simulink model "gm_spike_detection"  (R2020a)
settings: Solver=FixedStepDiscrete  StartTime=0.0  StopTime=840000  RelTol=1e-3
undefined symbols (not defined in the file or in its folder): Newton, Raphson
libraries: hdlsllib x8, simulink x4
settings Model: FPTRunName=FPA_Reference  PacingRate=40  Creator=BuccelliLab  LastModifiedBy=diflo
settings SolverCC: AutoInsertRateTranBlk=on  MinimalZcImpactIntegration=on
settings DataIOCC: LimitDataPoints=on  SaveOutput=off  SaveTime=off  ReturnWorkspaceOutputs=off
settings OptimizationCC: BlockReduction=off  ConditionallyExecuteInputs=off  DefaultParameterBehavior=Inlined  LifeSpan=inf
settings DebuggingCC: SignalRangeChecking=warning  ReadBeforeWriteMsg=DisableAll  WriteAfterWriteMsg=DisableAll  WriteAfterReadMsg=DisableAll  AlgebraicLoopMsg=error  InheritedTsInSrcMsg=none  MultiTaskDSMMsg=none  SingleTaskRateTransMsg=error  ParameterDowncastMsg=warning  ParameterOverflowMsg=warning  AllowSymbolicDim=off  StrictBusMsg=ErrorOnBusTreatedAsVector  SFUnexpectedBacktrackingDiag=warning  SFNoUnconditionalDefaultTransitionDiag=warning  SFExecutionAtInitializationDiag=none  ArithmeticOperatorsInVariantConditions=warning
settings HardwareCC: ProdBitPerPointer=32  ProdBitPerSizeT=32  ProdBitPerPtrDiffT=32  ProdLargestAtomicFloat=None  ProdIntDivRoundTo=Undefined  ProdEndianess=Unspecified  ProdWordSize=32  ProdHWDeviceType=ASIC/FPGA->ASIC/FPGA  TargetBitPerPointer=64  TargetBitPerSizeT=64  TargetBitPerPtrDiffT=64  TargetLongLongMode=on  TargetIntDivRoundTo=Zero  TargetEndianess=LittleEndian  TargetWordSize=64  TargetHWDeviceType=Custom Processor->MATLAB Host Computer  ProdEqTarget=off
settings ModelReferenceCC: UpdateModelReferenceTargets=IfOutOfDate
settings SFSimCC: SFSimEcho=off  SimUseLocalCustomCode=off  CustomCodeUndefinedFunction=UseInterfaceOnly
settings RTWCC: RTWUseLocalCustomCode=off
settings CodeAppCC: StateflowObjectComments=on
settings GRTTargetCC: TargetLangStandard=C89/C90 (ANSI)
settings ConfigComp: CovScope=ReferencedModels  CovMetricSettings=dw  CovHtmlReporting=on  CovSaveCumulativeToWorkspaceVar=on  CovSaveSingleToWorkspaceVar=on  CovExternalEMLEnable=off  CovSFcnEnable=off

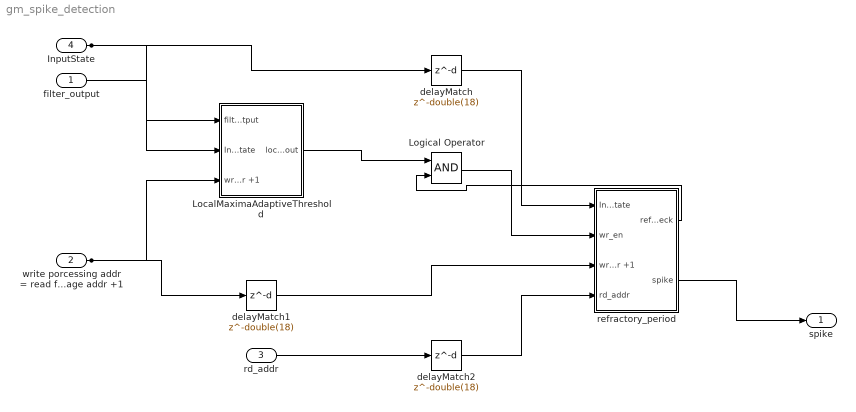
== system gm_spike_detection ==
  filter_output : Inport  OutDataTypeStr=uint16  PortDimensions=1  SampleTime=1
  write porcessing addr = read from storage addr +1 : Inport  Port=2  OutDataTypeStr=fixdt(0, 9, 0)  PortDimensions=1  SampleTime=1
  rd_addr : Inport  Port=3  OutDataTypeStr=fixdt(0, 9, 0)  PortDimensions=1  SampleTime=1
  InputState : Inport  Port=4  OutDataTypeStr=boolean  PortDimensions=1  SampleTime=1
  LocalMaximaAdaptiveThreshold : Subsystem
  Logical Operator : Logic  AllPortsSameDT=off  OutDataTypeStr=boolean  SampleTime=1
  delayMatch : Delay  DelayLength=double(18)  InitialCondition=0  SampleTime=1
  delayMatch1 : Delay  DelayLength=double(18)  InitialCondition=0  SampleTime=1
  delayMatch2 : Delay  DelayLength=double(18)  InitialCondition=0  SampleTime=1
  refractory_period : Subsystem
  spike : Outport  OutDataTypeStr=uint16  PortDimensions=1  SampleTime=[1,0]
  wires:
  filter_output/1 -> LocalMaximaAdaptiveThreshold/1(filter_output)
  delayMatch1/1 -> refractory_period/3(write porcessing addr = read from storage addr +1)
  delayMatch2/1 -> refractory_period/4(rd_addr)
  delayMatch/1 -> refractory_period/1(InputState)
  LocalMaximaAdaptiveThreshold/1(local_maxima_out) -> Logical Operator/1
  InputState/1 -> delayMatch/1, LocalMaximaAdaptiveThreshold/2(InputState)
  write porcessing addr = read from storage addr +1/1 -> delayMatch1/1, LocalMaximaAdaptiveThreshold/3(write porcessing addr = read from storage addr +1)
  rd_addr/1 -> delayMatch2/1
  Logical Operator/1 -> refractory_period/2(wr_en)
  refractory_period/1(refractory_check) -> Logical Operator/2
  refractory_period/2(spike) -> spike/1

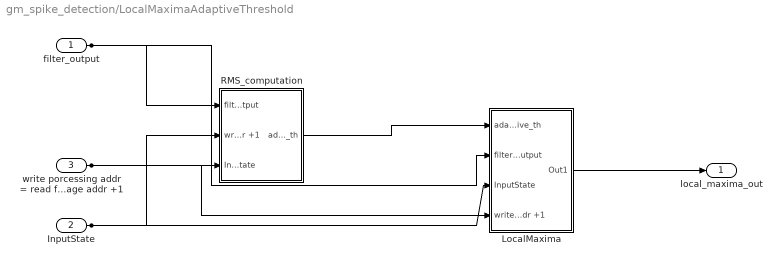
== system gm_spike_detection/LocalMaximaAdaptiveThreshold ==
  filter_output : Inport  OutDataTypeStr=uint16  PortDimensions=1  SampleTime=1
  InputState : Inport  Port=2  OutDataTypeStr=boolean  PortDimensions=1  SampleTime=1
  write porcessing addr = read from storage addr +1 : Inport  Port=3  OutDataTypeStr=fixdt(0, 9, 0)  PortDimensions=1  SampleTime=1
  LocalMaxima : Subsystem
  RMS_computation : Subsystem
  local_maxima_out : Outport
  wires:
  LocalMaxima/1(Out1) -> local_maxima_out/1
  RMS_computation/1(adaptive_th) -> LocalMaxima/1(adaptive_th)
  filter_output/1 -> LocalMaxima/2(filter_output), RMS_computation/1(filter_output)
  InputState/1 -> LocalMaxima/3(InputState), RMS_computation/3(InputState)
  write porcessing addr = read from storage addr +1/1 -> LocalMaxima/4(write porcessing addr = read from storage addr +1), RMS_computation/2(write porcessing addr = read from storage addr +1)

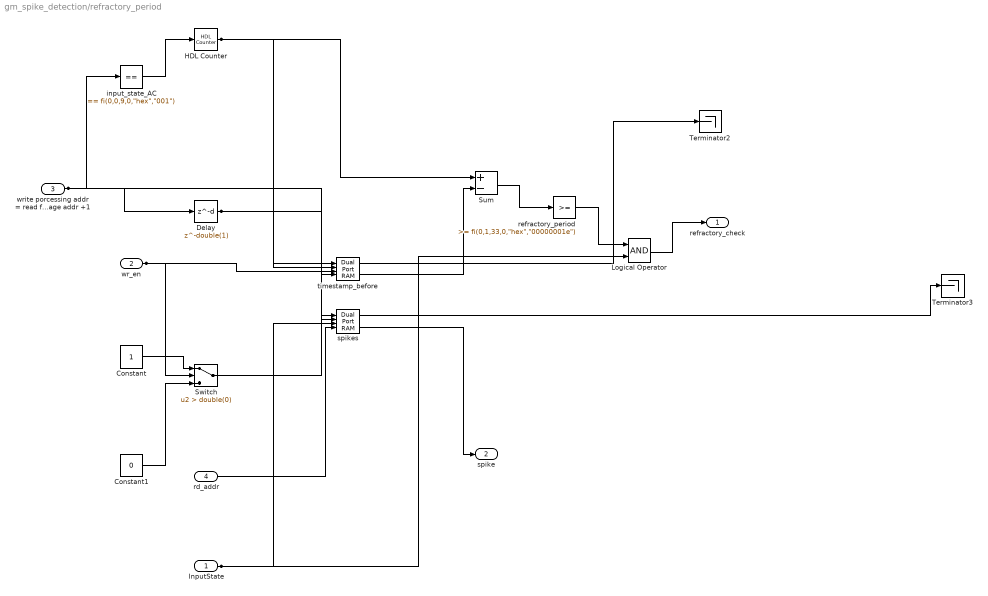
== system gm_spike_detection/refractory_period ==
  InputState : Inport  OutDataTypeStr=boolean  PortDimensions=1  SampleTime=1
  wr_en : Inport  Port=2  OutDataTypeStr=boolean  PortDimensions=1  SampleTime=1
  write porcessing addr = read from storage addr +1 : Inport  Port=3  OutDataTypeStr=fixdt(0, 9, 0)  PortDimensions=1  SampleTime=1
  rd_addr : Inport  Port=4  OutDataTypeStr=fixdt(0, 9, 0)  PortDimensions=1  SampleTime=1
  Constant : Constant  OutDataTypeStr=uint16  SampleTime=1
  Constant1 : Constant  Value=0  OutDataTypeStr=uint16  SampleTime=1
  Delay : Delay  DelayLength=double(1)  InitialCondition=0  SampleTime=1
  HDL Counter : hdlsllib/Sources/HDL Counter  CountType=Free running  CountInit=double(0)  CountStep=double(1)  CountMax=25  CountFromType=Initial value  CountFrom=double(0)  CountResetPort=off  CountLoadPort=off  CountEnbPort=on  CountDirPort=off  CountDataType=Unsigned  CountWordLen=32  CountFracLen=0  CountSampTime=1
  Logical Operator : Logic  AllPortsSameDT=off  OutDataTypeStr=boolean  SampleTime=1
  Sum : Sum  Inputs=+-  AccumDataTypeStr=fixdt(1, 33, 0)  OutDataTypeStr=fixdt(1, 33, 0)  SampleTime=1
  Switch : Switch  Criteria=u2 > Threshold  Threshold=double(0)  OutDataTypeStr=uint16  SampleTime=1
  Terminator2 : Terminator
  Terminator3 : Terminator
  input_state_AC : simulink/Logic and Bit Operations/Compare To Constant  relop===  const="fi(0,0,9,0,\"hex\",\"001\")"  OutDataTypeStr=boolean
  refractory_period : simulink/Logic and Bit Operations/Compare To Constant  relop=>=  const="fi(0,1,33,0,\"hex\",\"00000001e\")"  OutDataTypeStr=boolean
  spikes : hdlsllib/HDL RAMs/Dual Port RAM  ram_size=9
      settings: SourceProductBaseCode=SL
  timestamp_before : hdlsllib/HDL RAMs/Dual Port RAM  ram_size=9
      settings: SourceProductBaseCode=SL
  refractory_check : Outport
  spike : Outport  Port=2
  wires:
  InputState/1 -> Logical Operator/2, spikes/3
  wr_en/1 -> Switch/2, timestamp_before/3
  write porcessing addr = read from storage addr +1/1 -> input_state_AC/1, Delay/1, timestamp_before/4
  rd_addr/1 -> spikes/4
  Constant/1 -> Switch/1
  Constant1/1 -> Switch/3
  Delay/1 -> spikes/2, timestamp_before/2
  HDL Counter/1 -> Sum/1, timestamp_before/1
  Logical Operator/1 -> refractory_check/1
  Sum/1 -> refractory_period/1
  Switch/1 -> spikes/1
  input_state_AC/1 -> HDL Counter/1
  refractory_period/1 -> Logical Operator/1
  spikes/1 -> Terminator3/1
  spikes/2 -> spike/1
  timestamp_before/1 -> Terminator2/1
  timestamp_before/2 -> Sum/2

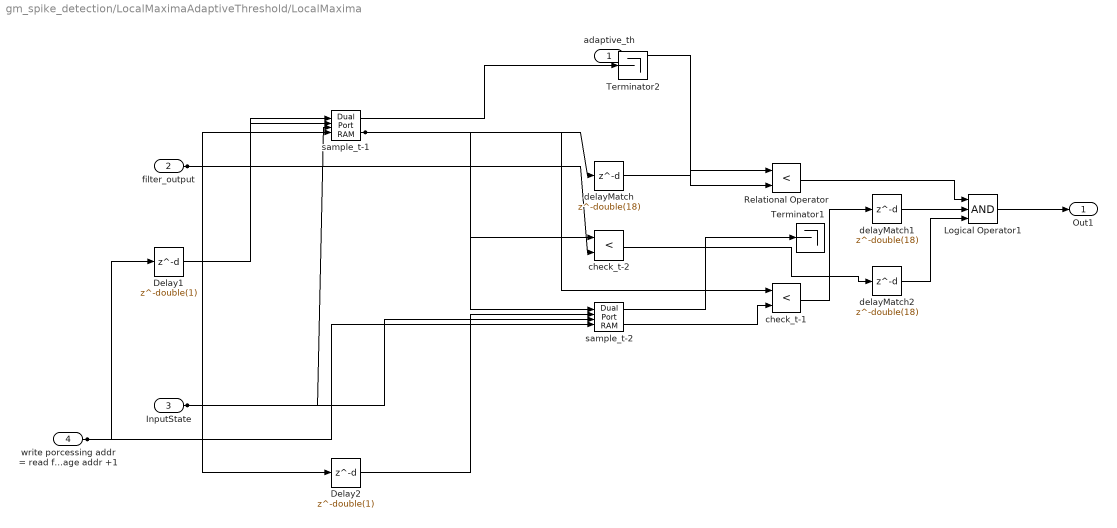
== system gm_spike_detection/LocalMaximaAdaptiveThreshold/LocalMaxima ==
  adaptive_th : Inport  OutDataTypeStr=uint16  PortDimensions=1  SampleTime=1
  filter_output : Inport  Port=2  OutDataTypeStr=uint16  PortDimensions=1  SampleTime=1
  InputState : Inport  Port=3  OutDataTypeStr=boolean  PortDimensions=1  SampleTime=1
  write porcessing addr = read from storage addr +1 : Inport  Port=4  OutDataTypeStr=fixdt(0, 9, 0)  PortDimensions=1  SampleTime=1
  Delay1 : Delay  DelayLength=double(1)  InitialCondition=0  SampleTime=1
  Delay2 : Delay  DelayLength=double(1)  InitialCondition=0  SampleTime=1
  Logical Operator1 : Logic  Inputs=3  AllPortsSameDT=off  OutDataTypeStr=boolean  SampleTime=1
  Relational Operator : RelationalOperator  Operator=<  OutDataTypeStr=boolean  SampleTime=1  RndMeth=Nearest
  Terminator1 : Terminator
  Terminator2 : Terminator
  check_t-1 : RelationalOperator  Operator=<  OutDataTypeStr=boolean  SampleTime=1  RndMeth=Nearest
  check_t-2 : RelationalOperator  Operator=<  OutDataTypeStr=boolean  SampleTime=1  RndMeth=Nearest
  delayMatch : Delay  DelayLength=double(18)  InitialCondition=0  SampleTime=1
  delayMatch1 : Delay  DelayLength=double(18)  InitialCondition=0  SampleTime=1
  delayMatch2 : Delay  DelayLength=double(18)  InitialCondition=0  SampleTime=1
  sample_t-1 : hdlsllib/HDL RAMs/Dual Port RAM  ram_size=9
      settings: SourceProductBaseCode=SL
  sample_t-2 : hdlsllib/HDL RAMs/Dual Port RAM  ram_size=9
      settings: SourceProductBaseCode=SL
  Out1 : Outport
  wires:
  Delay1/1 -> sample_t-1/2
  Delay2/1 -> sample_t-2/2
  Logical Operator1/1 -> Out1/1
  Relational Operator/1 -> Logical Operator1/1
  delayMatch1/1 -> Logical Operator1/2
  delayMatch2/1 -> Logical Operator1/3
  sample_t-1/1 -> Terminator2/1
  delayMatch/1 -> Relational Operator/1
  sample_t-2/1 -> Terminator1/1
  sample_t-2/2 -> check_t-1/2
  adaptive_th/1 -> Relational Operator/2
  filter_output/1 -> check_t-2/2, sample_t-1/1
  InputState/1 -> sample_t-1/3, sample_t-2/3
  write porcessing addr = read from storage addr +1/1 -> Delay2/1, Delay1/1, sample_t-1/4, sample_t-2/4
  sample_t-1/2 -> delayMatch/1, check_t-2/1, check_t-1/1, sample_t-2/1
  check_t-1/1 -> delayMatch1/1
  check_t-2/1 -> delayMatch2/1

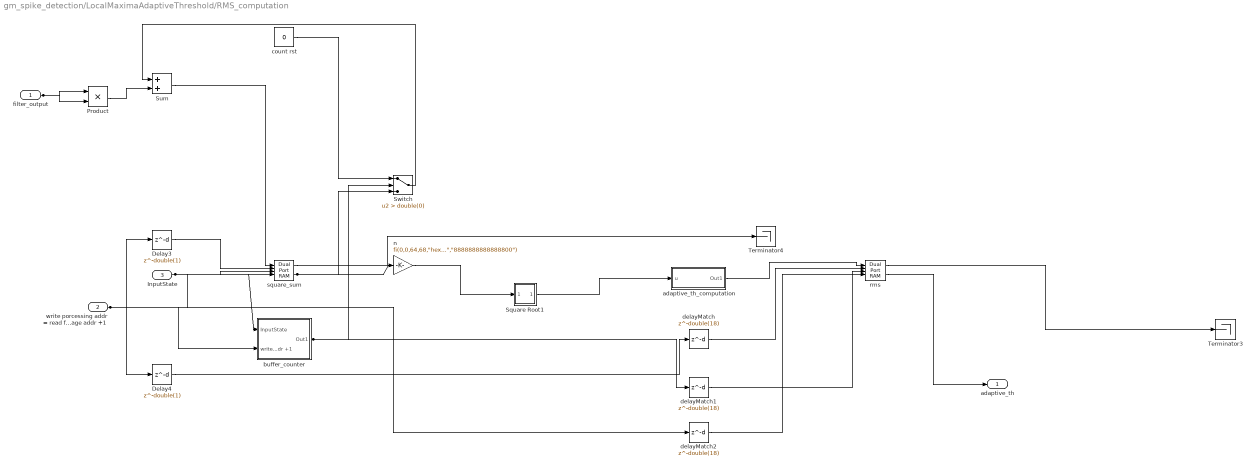
== system gm_spike_detection/LocalMaximaAdaptiveThreshold/RMS_computation ==
  filter_output : Inport  OutDataTypeStr=uint16  PortDimensions=1  SampleTime=1
  write porcessing addr = read from storage addr +1 : Inport  Port=2  OutDataTypeStr=fixdt(0, 9, 0)  PortDimensions=1  SampleTime=1
  InputState : Inport  Port=3  OutDataTypeStr=boolean  PortDimensions=1  SampleTime=1
  Delay3 : Delay  DelayLength=double(1)  InitialCondition=0  SampleTime=1
  Delay4 : Delay  DelayLength=double(1)  InitialCondition=0  SampleTime=1
  Product : Product  Inputs=**  OutDataTypeStr=uint32  SampleTime=1
  Square Root1 : Subsystem
  Sum : Sum  AccumDataTypeStr=fixdt(0, 65, 0)  OutDataTypeStr=fixdt(0, 64, 0)  SampleTime=1
  Switch : Switch  Criteria=u2 > Threshold  Threshold=double(0)  OutDataTypeStr=fixdt(0, 64, 0)  SampleTime=1
  Terminator3 : Terminator
  Terminator4 : Terminator
  adaptive_th_computation : Subsystem
  buffer_counter : Subsystem
  count rst : Constant  Value=0  OutDataTypeStr=fixdt(0, 64, 0)  SampleTime=1
  delayMatch : Delay  DelayLength=double(18)  InitialCondition=0  SampleTime=1
  delayMatch1 : Delay  DelayLength=double(18)  InitialCondition=0  SampleTime=1
  delayMatch2 : Delay  DelayLength=double(18)  InitialCondition=0  SampleTime=1
  n : Gain  Gain="fi(0,0,64,68,\"hex\",\"8888888888888800\")"  ParamDataTypeStr=fixdt(0, 64, 68)  OutDataTypeStr=fixdt(0, 40, 0)  SampleTime=1
  rms : hdlsllib/HDL RAMs/Dual Port RAM  ram_size=9
      settings: SourceProductBaseCode=SL
  square_sum : hdlsllib/HDL RAMs/Dual Port RAM  ram_size=9
      settings: SourceProductBaseCode=SL
  adaptive_th : Outport
  wires:
  delayMatch2/1 -> rms/4
  Delay3/1 -> square_sum/2
  delayMatch/1 -> rms/2
  Product/1 -> Sum/2
  Square Root1/1(Out1) -> adaptive_th_computation/1(u)
  adaptive_th_computation/1(Out1) -> rms/1
  delayMatch1/1 -> rms/3
  count rst/1 -> Switch/1
  n/1 -> Square Root1/1(In1)
  rms/1 -> Terminator3/1
  rms/2 -> adaptive_th/1
  square_sum/1 -> Terminator4/1
  square_sum/2 -> n/1, Switch/3
  filter_output/1 -> Product/2, Product/1
  write porcessing addr = read from storage addr +1/1 -> delayMatch2/1, Delay4/1, Delay3/1, buffer_counter/2(write porcessing addr = read from storage addr +1), square_sum/4
  InputState/1 -> buffer_counter/1(InputState), square_sum/3
  Delay4/1 -> delayMatch/1
  buffer_counter/1(Out1) -> delayMatch1/1, Switch/2
  Sum/1 -> square_sum/1
  Switch/1 -> Sum/1

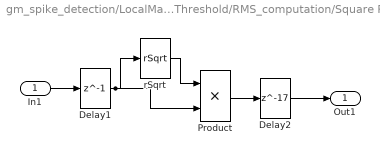
== system gm_spike_detection/LocalMaximaAdaptiveThreshold/RMS_computation/Square Root1 ==
  In1 : Inport
  Delay1 : Delay  DelayLength=1
  Delay2 : Delay  DelayLength=17
  Product : Product  OutDataTypeStr=uint16  SaturateOnIntegerOverflow=on
  rSqrt : Sqrt  Operator=rSqrt  OutDataTypeStr=fixdt(0,40,40)  RndMeth=Nearest  IntermediateResultsDataTypeStr=Inherit: Inherit from output  AlgorithmType=Newton-Raphson  SaturateOnIntegerOverflow=on
  Out1 : Outport
  wires:
  In1/1 -> Delay1/1
  Delay1/1 -> rSqrt/1, Product/2
  rSqrt/1 -> Product/1
  Product/1 -> Delay2/1
  Delay2/1 -> Out1/1

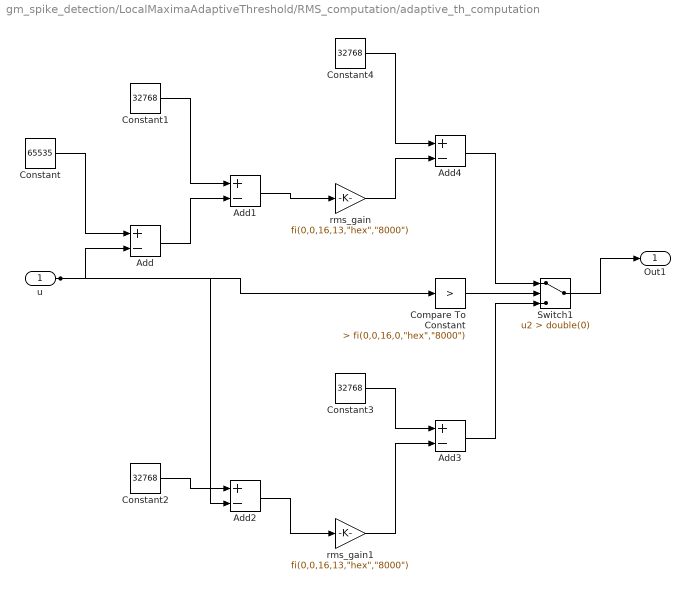
== system gm_spike_detection/LocalMaximaAdaptiveThreshold/RMS_computation/adaptive_th_computation ==
  u : Inport  OutDataTypeStr=uint16  PortDimensions=1  SampleTime=1
  Add{,1..4} (5 alike) : Sum  Inputs=+-  AccumDataTypeStr=uint16  OutDataTypeStr=uint16  SampleTime=1
  Compare To Constant : simulink/Logic and Bit Operations/Compare To Constant  relop=>  const="fi(0,0,16,0,\"hex\",\"8000\")"  OutDataTypeStr=boolean
  Constant : Constant  Value=65535  OutDataTypeStr=uint16  SampleTime=1
  Constant{1..4} (4 alike) : Constant  Value=32768  OutDataTypeStr=uint16  SampleTime=1
  Switch1 : Switch  Criteria=u2 > Threshold  Threshold=double(0)  OutDataTypeStr=uint16  SampleTime=1
  rms_gain : Gain  Gain="fi(0,0,16,13,\"hex\",\"8000\")"  ParamDataTypeStr=fixdt(0, 16, 13)  OutDataTypeStr=uint16  SampleTime=1
  rms_gain1 : Gain  Gain="fi(0,0,16,13,\"hex\",\"8000\")"  ParamDataTypeStr=fixdt(0, 16, 13)  OutDataTypeStr=uint16  SampleTime=1
  Out1 : Outport
  wires:
  Add/1 -> Add1/2
  Add1/1 -> rms_gain/1
  Add2/1 -> rms_gain1/1
  Add3/1 -> Switch1/3
  Add4/1 -> Switch1/1
  Compare To Constant/1 -> Switch1/2
  Constant/1 -> Add/1
  Constant1/1 -> Add1/1
  Constant2/1 -> Add2/1
  Constant3/1 -> Add3/1
  Constant4/1 -> Add4/1
  Switch1/1 -> Out1/1
  rms_gain/1 -> Add4/2
  rms_gain1/1 -> Add3/2
  u/1 -> Compare To Constant/1, Add2/2, Add/2

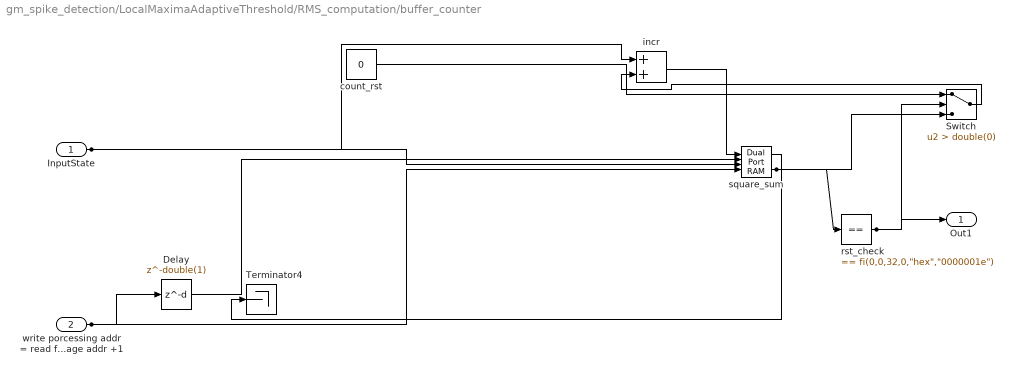
== system gm_spike_detection/LocalMaximaAdaptiveThreshold/RMS_computation/buffer_counter ==
  InputState : Inport  OutDataTypeStr=boolean  PortDimensions=1  SampleTime=1
  write porcessing addr = read from storage addr +1 : Inport  Port=2  OutDataTypeStr=fixdt(0, 9, 0)  PortDimensions=1  SampleTime=1
  Delay : Delay  DelayLength=double(1)  InitialCondition=0  SampleTime=1
  Switch : Switch  Criteria=u2 > Threshold  Threshold=double(0)  OutDataTypeStr=uint32  SampleTime=1
  Terminator4 : Terminator
  count_rst : Constant  Value=0  OutDataTypeStr=uint16  SampleTime=1
  incr : Sum  AccumDataTypeStr=uint32  OutDataTypeStr=uint32  SampleTime=1
  rst_check : simulink/Logic and Bit Operations/Compare To Constant  relop===  const="fi(0,0,32,0,\"hex\",\"0000001e\")"  OutDataTypeStr=boolean
  square_sum : hdlsllib/HDL RAMs/Dual Port RAM  ram_size=9
      settings: SourceProductBaseCode=SL
  Out1 : Outport
  wires:
  Delay/1 -> square_sum/2
  count_rst/1 -> Switch/1
  rst_check/1 -> Out1/1, Switch/2
  square_sum/1 -> Terminator4/1
  InputState/1 -> incr/1, square_sum/3
  write porcessing addr = read from storage addr +1/1 -> Delay/1, square_sum/4
  incr/1 -> square_sum/1
  Switch/1 -> incr/2
  square_sum/2 -> rst_check/1, Switch/3
